simulink model "BR"  (R2020b)
settings: Solver=VariableStepAuto  StartTime=0.0  StopTime=10  RelTol=1e-3
undefined symbols (not defined in the file): U_nom
libraries: dspstat3 x12, powerlib x12, powerlib_meascontrol x3
settings Model: Creator=New-life  LastModifiedBy=New-life

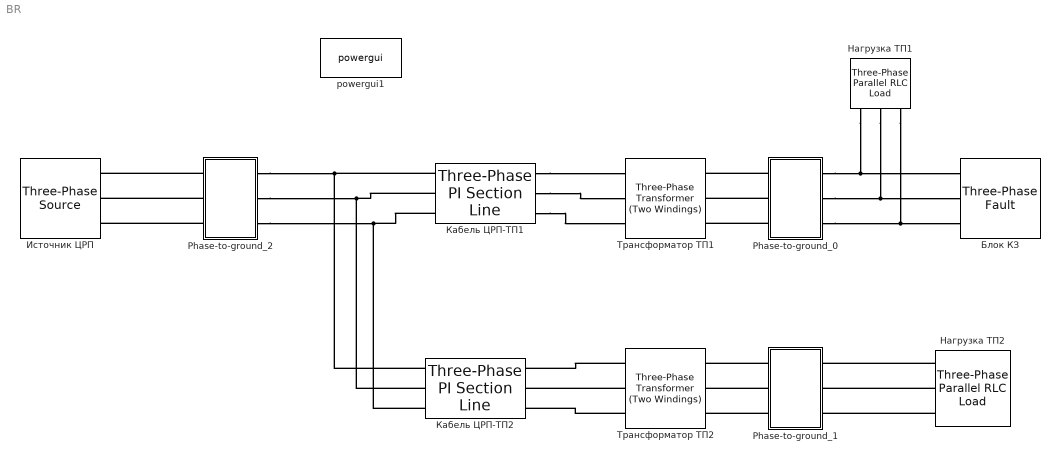
== system BR ==
  Phase-to-ground_0 : Subsystem
      settings: CopyFcn=|
      | % Получаем путь и имя нового (только что скопированного) блока
      | blockPath = gcb;
      | blockName = get_param(blockPath, 'Name');
      | 
      | % Ищем число в названии самой подсистемы (например, берем "2" из "Measure_2")
      | numStr = regexp(blockName, '\d+', 'match');
      | 
      | if ~isempty(numStr)
      |     newNum = numStr{end}; % Берем последнее найденное число
      | 
      |     % --- 1. Обновляем скрытые теги в Goto и From (радиочастоты) ---
      |     gotos = find_system(blockPath, 'LookUnderMasks', 'on', 'BlockType', 'Goto');
      |     froms = find_system(blockPath, 'LookUnderMasks', 'on', 'BlockType', 'From');
      | 
      |     for i = 1:length(gotos)
      |         oldTag = get_param(gotos{i}, 'GotoTag');
      |         set_param(gotos{i}, 'GotoTag', regexprep(oldTag, '\d+$', newNum));
      |     end
      |     for i = 1:length(froms)
      |         oldTag = get_param(froms{i}, 'GotoTag');
      |         set_param(froms{i}, 'GotoTag', regexprep(oldTag, '\d+$', newNum));
      |     end
      | 
      |     % --- 2. ПЕРЕИМЕНОВЫВАЕМ САМИ БЛОКИ (визуальные надписи UI0 -> UI1 и т.д.) ---
      |     % Ищем все элементы только внутри этой подсистемы
      |     internalBlocks = find_system(blockPath, 'SearchDepth', 1, 'LookUnderMasks', 'on');
      | 
      |     % Цикл начинаем с 2, так как 1-й элемент в списке - это сама папка подсистемы
      |     for i = 2:length(internalBlocks)
      |         oldName = get_param(internalBlocks{i}, 'Name');
      |         % Ищем цифру в конце имени и меняем на новую
      |         newName = regexprep(oldName, '\d+$', newNum);
      | 
      |         % Если имя изменилось, применяем его
      |         if ~strcmp(oldName, newName)
      |             try
      |                 set_param(internalBlocks{i}, 'Name', newName);
      |             catch
      |                 % Игнорируем ошибку, если вдруг такое имя уже случайно есть
      |             end
      |         end
      |     end
      | end
  Phase-to-ground_1 : Subsystem
      settings: CopyFcn=|
      | % Получаем путь и имя нового (только что скопированного) блока
      | blockPath = gcb;
      | blockName = get_param(blockPath, 'Name');
      | 
      | % Ищем число в названии самой подсистемы (например, берем "2" из "Measure_2")
      | numStr = regexp(blockName, '\d+', 'match');
      | 
      | if ~isempty(numStr)
      |     newNum = numStr{end}; % Берем последнее найденное число
      | 
      |     % --- 1. Обновляем скрытые теги в Goto и From (радиочастоты) ---
      |     gotos = find_system(blockPath, 'LookUnderMasks', 'on', 'BlockType', 'Goto');
      |     froms = find_system(blockPath, 'LookUnderMasks', 'on', 'BlockType', 'From');
      | 
      |     for i = 1:length(gotos)
      |         oldTag = get_param(gotos{i}, 'GotoTag');
      |         set_param(gotos{i}, 'GotoTag', regexprep(oldTag, '\d+$', newNum));
      |     end
      |     for i = 1:length(froms)
      |         oldTag = get_param(froms{i}, 'GotoTag');
      |         set_param(froms{i}, 'GotoTag', regexprep(oldTag, '\d+$', newNum));
      |     end
      | 
      |     % --- 2. ПЕРЕИМЕНОВЫВАЕМ САМИ БЛОКИ (визуальные надписи UI0 -> UI1 и т.д.) ---
      |     % Ищем все элементы только внутри этой подсистемы
      |     internalBlocks = find_system(blockPath, 'SearchDepth', 1, 'LookUnderMasks', 'on');
      | 
      |     % Цикл начинаем с 2, так как 1-й элемент в списке - это сама папка подсистемы
      |     for i = 2:length(internalBlocks)
      |         oldName = get_param(internalBlocks{i}, 'Name');
      |         % Ищем цифру в конце имени и меняем на новую
      |         newName = regexprep(oldName, '\d+$', newNum);
      | 
      |         % Если имя изменилось, применяем его
      |         if ~strcmp(oldName, newName)
      |             try
      |                 set_param(internalBlocks{i}, 'Name', newName);
      |             catch
      |                 % Игнорируем ошибку, если вдруг такое имя уже случайно есть
      |             end
      |         end
      |     end
      | end
  Phase-to-ground_2 : Subsystem
      settings: CopyFcn=|
      | % Получаем путь и имя нового (только что скопированного) блока
      | blockPath = gcb;
      | blockName = get_param(blockPath, 'Name');
      | 
      | % Ищем число в названии самой подсистемы (например, берем "2" из "Measure_2")
      | numStr = regexp(blockName, '\d+', 'match');
      | 
      | if ~isempty(numStr)
      |     newNum = numStr{end}; % Берем последнее найденное число
      | 
      |     % --- 1. Обновляем скрытые теги в Goto и From (радиочастоты) ---
      |     gotos = find_system(blockPath, 'LookUnderMasks', 'on', 'BlockType', 'Goto');
      |     froms = find_system(blockPath, 'LookUnderMasks', 'on', 'BlockType', 'From');
      | 
      |     for i = 1:length(gotos)
      |         oldTag = get_param(gotos{i}, 'GotoTag');
      |         set_param(gotos{i}, 'GotoTag', regexprep(oldTag, '\d+$', newNum));
      |     end
      |     for i = 1:length(froms)
      |         oldTag = get_param(froms{i}, 'GotoTag');
      |         set_param(froms{i}, 'GotoTag', regexprep(oldTag, '\d+$', newNum));
      |     end
      | 
      |     % --- 2. ПЕРЕИМЕНОВЫВАЕМ САМИ БЛОКИ (визуальные надписи UI0 -> UI1 и т.д.) ---
      |     % Ищем все элементы только внутри этой подсистемы
      |     internalBlocks = find_system(blockPath, 'SearchDepth', 1, 'LookUnderMasks', 'on');
      | 
      |     % Цикл начинаем с 2, так как 1-й элемент в списке - это сама папка подсистемы
      |     for i = 2:length(internalBlocks)
      |         oldName = get_param(internalBlocks{i}, 'Name');
      |         % Ищем цифру в конце имени и меняем на новую
      |         newName = regexprep(oldName, '\d+$', newNum);
      | 
      |         % Если имя изменилось, применяем его
      |         if ~strcmp(oldName, newName)
      |             try
      |                 set_param(internalBlocks{i}, 'Name', newName);
      |             catch
      |                 % Игнорируем ошибку, если вдруг такое имя уже случайно есть
      |             end
      |         end
      |     end
      | end
  powergui1 : powerlib/powergui  Priority=1  SimulationMode=Discrete  SampleTime=5e-5  frequency=60  Iterations=50  frequencyindice=50  Pbase=100e6  ErrMax=1e-4  UnitsV=kV  UnitsW=MW  buscounter=0  FunctionMessages=off  echomessages=off  EnableUseOfTLC=off  CurrentSourceSwitches=off  DisableSnubberDevices=off  DisableRonSwitches=off  DisableVfSwitches=off  DisplayEquations=off  AutomaticDiscreteSolvers=off  SolverType=Tustin/Backward Euler (TBE)  Interpol=off  ExternalGateDelay=off  methode=off  Ts=100  x0status=blocks  SPID=on  SwTol=0  HookPort=off  NonlinearTolerance=1e-4  nMaxIteration=100  ContinueOnMaxIteration=off  RestoreLinks=warning  ResistiveCurrentMeasurement=off  Frange=[0:2:500]  Ylog=off  Xlog=on  ShowGrid=off  save=off  variable=ZData  structure=0  ZoomFFT=off  StartTime=0.0  cycles=1  DisplayStyle=1  fundamental=60  FreqAxis=off  MaxFrequency=1000  frequencyindicesteady=1  RmsSteady=1  display=off
  Блок КЗ : powerlib/Elements/Three-Phase Fault  InitialStates=0  FaultA=on  FaultB=on  FaultC=on  GroundFault=off  SwitchTimes=T_fault  External=off  SwitchStatus=NaN  FaultResistance=0.001  GroundResistance=0.01  SnubberResistance=1e6  SnubberCapacitance=inf  Measurements=None
  Источник ЦРП : powerlib/Electrical Sources/Three-Phase Source  InternalConnection=Yg  VoltagePhases=off  Voltage=U_nom  PhaseAngle=0  Voltage_phases=[25e3 25e3 25e3]/sqrt(3)  PhaseAngles_phases=[0 -120 +120]  Frequency=50  NonIdealSource=on  SpecifyImpedance=on  Resistance=0.8929  Inductance=16.58e-3  ShortCircuitLevel=S_kz_sys  BaseVoltage=U_nom  XRratio=7  BusType=swing  Pref=10e3  Qref=0  Prefabc=[10e3, 10e3, 10e3]  Qrefabc=[0, 0, 0]  Qmin=-inf  Qmax=inf
  Кабель ЦРП-ТП1 : powerlib/Elements/Three-Phase PI Section Line  LConnTagsString=a|b|c  RConnTagsString=A|B|C  Length=L_cab1  Frequency=60  Resistances=[0.3 0.3]  Inductances=[0.637e-3 0.637e-3]  Capacitances=[0.3e-6 0.3e-6]
  Кабель ЦРП-ТП2 : powerlib/Elements/Three-Phase PI Section Line  LConnTagsString=a|b|c  RConnTagsString=A|B|C  Length=L_cab2  Frequency=60  Resistances=[0.3 0.3]  Inductances=[0.637e-3 0.637e-3]  Capacitances=[0.3e-6 0.3e-6]
  Нагрузка ТП1 : powerlib/Elements/Three-Phase Parallel RLC Load  LConnTagsString=A|B|C  Configuration=Y (grounded)  NominalVoltage=400  Vabc=[1e3 1e3 1e3]  Vabcp=[1e3 1e3 1e3]  NominalFrequency=50  UnbalancedPower=off  ActivePower=P_t1  InductivePower=Q_t1  CapacitivePower=0  Pabc=[10e3 9e3 11e3]  QLabc=[100 90 110]  QCabc=[100 90 110]  Pabcp=[10e3 9e3 11e3]  QLabcp=[100 90 110]  QCabcp=[100 90 110]  Measurements=None  LoadType=constant Z
  Нагрузка ТП2 : powerlib/Elements/Three-Phase Parallel RLC Load  LConnTagsString=A|B|C  Configuration=Y (grounded)  NominalVoltage=400  Vabc=[1e3 1e3 1e3]  Vabcp=[1e3 1e3 1e3]  NominalFrequency=50  UnbalancedPower=off  ActivePower=P_t2  InductivePower=Q_t2  CapacitivePower=0  Pabc=[10e3 9e3 11e3]  QLabc=[100 90 110]  QCabc=[100 90 110]  Pabcp=[10e3 9e3 11e3]  QLabcp=[100 90 110]  QCabcp=[100 90 110]  Measurements=None  LoadType=constant Z
  Трансформатор ТП1 : powerlib/Elements/Three-Phase Transformer (Two Windings)  Winding1Connection=Yg  Winding2Connection=Yg  CoreType=Three single-phase transformers  SetSaturation=off  Hysteresis=off  DataFile='hysteresis'  SetInitialFlux=off  Measurements=None  UNITS=pu  NominalPower=[630e3 50]  Winding1=[6000 0.005 0.02]  Winding2=[400 0.005 0.02]  Rm=500  Lm=500  L0=0.5  Saturation=[ 0,0 ; 0.0024,1.2 ; 1.0,1.52 ]  InitialFluxes=[ 0.8 , -0.8 , 0.7 ]  BreakLoop=off  DiscreteSolver=Trapezoidal iterative  DataType=off  TransfoNumber=1
  Трансформатор ТП2 : powerlib/Elements/Three-Phase Transformer (Two Windings)  Winding1Connection=Yg  Winding2Connection=Yg  CoreType=Three single-phase transformers  SetSaturation=off  Hysteresis=off  DataFile='hysteresis'  SetInitialFlux=off  Measurements=None  UNITS=pu  NominalPower=[630e3 50]  Winding1=[6000 0.005 0.02]  Winding2=[400 0.005 0.02]  Rm=500  Lm=500  L0=0.5  Saturation=[ 0,0 ; 0.0024,1.2 ; 1.0,1.52 ]  InitialFluxes=[ 0.8 , -0.8 , 0.7 ]  BreakLoop=off  DiscreteSolver=Trapezoidal iterative  DataType=off  TransfoNumber=1
  connections:
  Кабель ЦРП-ТП1/LConn1 -- Phase-to-ground_2/RConn1 -- Кабель ЦРП-ТП2/LConn1
  Кабель ЦРП-ТП1/LConn3 -- Phase-to-ground_2/RConn3 -- Кабель ЦРП-ТП2/LConn3
  Кабель ЦРП-ТП1/LConn2 -- Phase-to-ground_2/RConn2 -- Кабель ЦРП-ТП2/LConn2
  Кабель ЦРП-ТП1/RConn2 -- Трансформатор ТП1/LConn2
  Кабель ЦРП-ТП1/RConn3 -- Трансформатор ТП1/LConn3
  Кабель ЦРП-ТП1/RConn1 -- Трансформатор ТП1/LConn1
  Phase-to-ground_0/LConn2 -- Трансформатор ТП1/RConn2
  Phase-to-ground_0/LConn1 -- Трансформатор ТП1/RConn1
  Phase-to-ground_0/LConn3 -- Трансформатор ТП1/RConn3
  Phase-to-ground_0/RConn1 -- Нагрузка ТП1/LConn1 -- Блок КЗ/LConn1
  Phase-to-ground_0/RConn2 -- Нагрузка ТП1/LConn2 -- Блок КЗ/LConn2
  Phase-to-ground_0/RConn3 -- Блок КЗ/LConn3 -- Нагрузка ТП1/LConn3
  Нагрузка ТП2/LConn1 -- Phase-to-ground_1/RConn1
  Нагрузка ТП2/LConn2 -- Phase-to-ground_1/RConn2
  Нагрузка ТП2/LConn3 -- Phase-to-ground_1/RConn3
  Phase-to-ground_1/LConn1 -- Трансформатор ТП2/RConn1
  Phase-to-ground_1/LConn2 -- Трансформатор ТП2/RConn2
  Phase-to-ground_1/LConn3 -- Трансформатор ТП2/RConn3
  Трансформатор ТП2/LConn1 -- Кабель ЦРП-ТП2/RConn1
  Трансформатор ТП2/LConn2 -- Кабель ЦРП-ТП2/RConn2
  Трансформатор ТП2/LConn3 -- Кабель ЦРП-ТП2/RConn3
  Phase-to-ground_2/LConn3 -- Источник ЦРП/RConn3
  Phase-to-ground_2/LConn2 -- Источник ЦРП/RConn2
  Phase-to-ground_2/LConn1 -- Источник ЦРП/RConn1

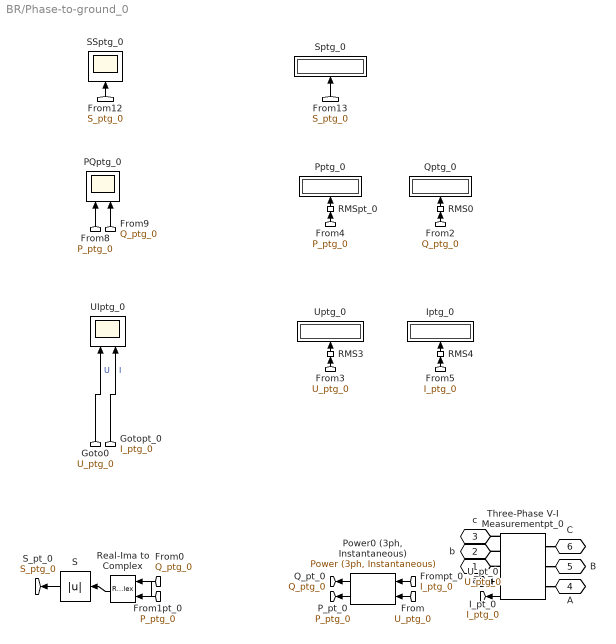
== system BR/Phase-to-ground_0 ==
  Iptg_0 : Display
      settings: Format=bank
  PQptg_0 : Scope  NumInputPorts=2
  "Power0 (3ph, Instantaneous)" : powerlib_meascontrol/Measurements/Power (3ph, Instantaneous)
  Pptg_0 : Display
      settings: Format=bank
  Qptg_0 : Display
      settings: Format=bank
  RMS0 : dspstat3/RMS  run=off  directionMode=Each column  dimension=1  InputProcessing=Columns as channels (frame based)  reset_popup=None
  RMS3 : dspstat3/RMS  run=off  directionMode=Each column  dimension=1  InputProcessing=Columns as channels (frame based)  reset_popup=None
  RMS4 : dspstat3/RMS  run=off  directionMode=Each column  dimension=1  InputProcessing=Columns as channels (frame based)  reset_popup=None
  RMSpt_0 : dspstat3/RMS  run=off  directionMode=Each column  dimension=1  InputProcessing=Columns as channels (frame based)  reset_popup=None
  Real-Ima to Complex : RealImagToComplex
  S : Abs
  SSptg_0 : Scope
  Sptg_0 : Display
      settings: Format=bank
  Three-Phase V-I Measurementpt_0 : powerlib/Measurements/Three-Phase V-I Measurement  VoltageMeasurement=phase-to-ground  SetLabelV=off  LabelV=Vabc  Vpu=off  VpuLL=off  CurrentMeasurement=yes  SetLabelI=off  LabelI=Iabc  Ipu=off  Pbase=100e6  Vbase=500e3  OutputType=Complex  PhasorSimulation=off  PSBequivalent=0
  UIptg_0 : Scope  NumInputPorts=2
  Uptg_0 : Display
      settings: Format=bank
  a : PMIOPort  Side=Right
  b : PMIOPort  Port=2  Side=Right
  c : PMIOPort  Port=3  Side=Right
  A : PMIOPort  Port=4  Side=Left
  B : PMIOPort  Port=5  Side=Left
  C : PMIOPort  Port=6  Side=Left
  tag scope: I_ptg_0=global, P_ptg_0=global, Q_ptg_0=global, S_ptg_0=global, U_ptg_0=global
  wires:
  S/1 -> [S_ptg_0]
  Real-Ima to Complex/1 -> S/1
  [S_ptg_0] -> Sptg_0/1
  [S_ptg_0] -> SSptg_0/1
  [P_ptg_0] -> RMSpt_0/1
  RMSpt_0/1 -> Pptg_0/1
  RMS0/1 -> Qptg_0/1
  [U_ptg_0] -> RMS3/1
  RMS3/1 -> Uptg_0/1
  [P_ptg_0] -> Real-Ima to Complex/1
  [Q_ptg_0] -> RMS0/1
  [I_ptg_0] -> RMS4/1
  RMS4/1 -> Iptg_0/1
  [P_ptg_0] -> PQptg_0/1
  [I_ptg_0] -> UIptg_0/2  "I"
  Three-Phase V-I Measurementpt_0/1 -> [U_ptg_0]
  [Q_ptg_0] -> Real-Ima to Complex/2
  Three-Phase V-I Measurementpt_0/2 -> [I_ptg_0]
  [U_ptg_0] -> "Power0 (3ph, Instantaneous)"/1
  [I_ptg_0] -> "Power0 (3ph, Instantaneous)"/2
  [Q_ptg_0] -> PQptg_0/2
  "Power0 (3ph, Instantaneous)"/2 -> [Q_ptg_0]
  "Power0 (3ph, Instantaneous)"/1 -> [P_ptg_0]
  [U_ptg_0] -> UIptg_0/1  "U"
  connections:
  Three-Phase V-I Measurementpt_0/LConn1 -- A/RConn1
  Three-Phase V-I Measurementpt_0/RConn1 -- a/RConn1
  Three-Phase V-I Measurementpt_0/LConn2 -- B/RConn1
  Three-Phase V-I Measurementpt_0/LConn3 -- C/RConn1
  Three-Phase V-I Measurementpt_0/RConn3 -- c/RConn1
  Three-Phase V-I Measurementpt_0/RConn2 -- b/RConn1

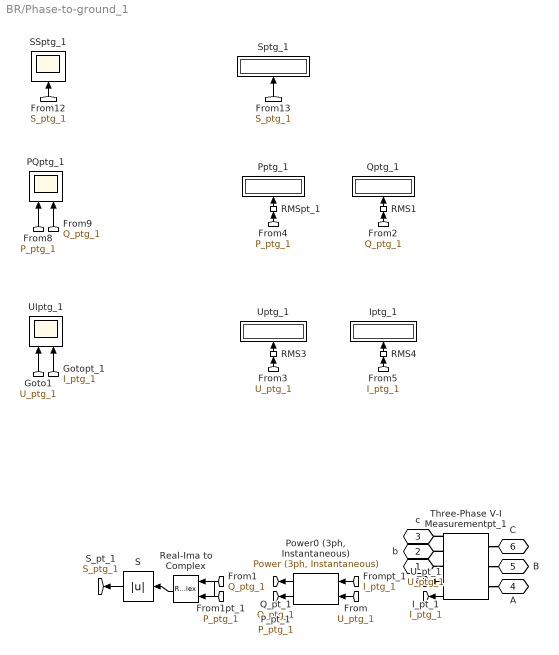
== system BR/Phase-to-ground_1 ==
  Iptg_1 : Display
      settings: Format=bank
  PQptg_1 : Scope  NumInputPorts=2
  "Power0 (3ph, Instantaneous)" : powerlib_meascontrol/Measurements/Power (3ph, Instantaneous)
  Pptg_1 : Display
      settings: Format=bank
  Qptg_1 : Display
      settings: Format=bank
  RMS1 : dspstat3/RMS  run=off  directionMode=Each column  dimension=1  InputProcessing=Columns as channels (frame based)  reset_popup=None
  RMS3 : dspstat3/RMS  run=off  directionMode=Each column  dimension=1  InputProcessing=Columns as channels (frame based)  reset_popup=None
  RMS4 : dspstat3/RMS  run=off  directionMode=Each column  dimension=1  InputProcessing=Columns as channels (frame based)  reset_popup=None
  RMSpt_1 : dspstat3/RMS  run=off  directionMode=Each column  dimension=1  InputProcessing=Columns as channels (frame based)  reset_popup=None
  Real-Ima to Complex : RealImagToComplex
  S : Abs
  SSptg_1 : Scope
  Sptg_1 : Display
      settings: Format=bank
  Three-Phase V-I Measurementpt_1 : powerlib/Measurements/Three-Phase V-I Measurement  VoltageMeasurement=phase-to-ground  SetLabelV=off  LabelV=Vabc  Vpu=off  VpuLL=off  CurrentMeasurement=yes  SetLabelI=off  LabelI=Iabc  Ipu=off  Pbase=100e6  Vbase=500e3  OutputType=Complex  PhasorSimulation=off  PSBequivalent=0
  UIptg_1 : Scope  NumInputPorts=2
  Uptg_1 : Display
      settings: Format=bank
  a : PMIOPort  Side=Right
  b : PMIOPort  Port=2  Side=Right
  c : PMIOPort  Port=3  Side=Right
  A : PMIOPort  Port=4  Side=Left
  B : PMIOPort  Port=5  Side=Left
  C : PMIOPort  Port=6  Side=Left
  tag scope: I_ptg_1=global, P_ptg_1=global, Q_ptg_1=global, S_ptg_1=global, U_ptg_1=global
  wires:
  [Q_ptg_1] -> PQptg_1/2
  "Power0 (3ph, Instantaneous)"/1 -> [P_ptg_1]
  "Power0 (3ph, Instantaneous)"/2 -> [Q_ptg_1]
  [I_ptg_1] -> "Power0 (3ph, Instantaneous)"/2
  [U_ptg_1] -> "Power0 (3ph, Instantaneous)"/1
  Three-Phase V-I Measurementpt_1/2 -> [I_ptg_1]
  [Q_ptg_1] -> Real-Ima to Complex/2
  Three-Phase V-I Measurementpt_1/1 -> [U_ptg_1]
  [I_ptg_1] -> UIptg_1/2
  [P_ptg_1] -> PQptg_1/1
  [U_ptg_1] -> UIptg_1/1
  RMS4/1 -> Iptg_1/1
  [I_ptg_1] -> RMS4/1
  [Q_ptg_1] -> RMS1/1
  [P_ptg_1] -> Real-Ima to Complex/1
  RMS3/1 -> Uptg_1/1
  [U_ptg_1] -> RMS3/1
  RMS1/1 -> Qptg_1/1
  RMSpt_1/1 -> Pptg_1/1
  [P_ptg_1] -> RMSpt_1/1
  [S_ptg_1] -> SSptg_1/1
  [S_ptg_1] -> Sptg_1/1
  Real-Ima to Complex/1 -> S/1
  S/1 -> [S_ptg_1]
  connections:
  Three-Phase V-I Measurementpt_1/RConn2 -- b/RConn1
  Three-Phase V-I Measurementpt_1/RConn3 -- c/RConn1
  Three-Phase V-I Measurementpt_1/LConn3 -- C/RConn1
  Three-Phase V-I Measurementpt_1/LConn2 -- B/RConn1
  Three-Phase V-I Measurementpt_1/RConn1 -- a/RConn1
  Three-Phase V-I Measurementpt_1/LConn1 -- A/RConn1

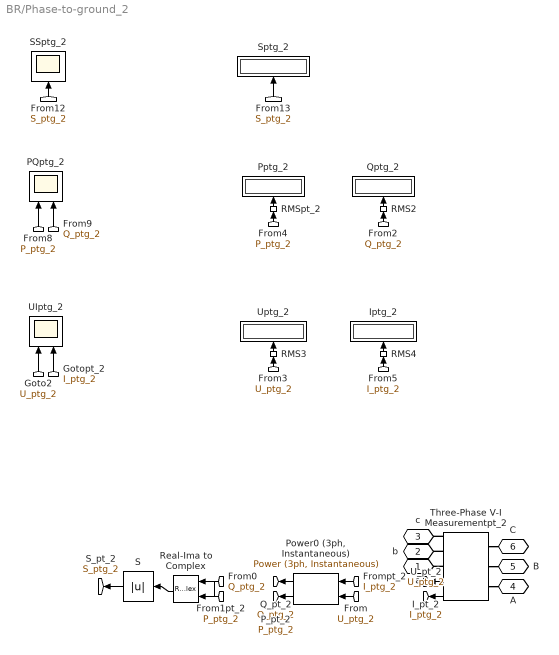
== system BR/Phase-to-ground_2 ==
  Iptg_2 : Display
      settings: Format=bank
  PQptg_2 : Scope  NumInputPorts=2
  "Power0 (3ph, Instantaneous)" : powerlib_meascontrol/Measurements/Power (3ph, Instantaneous)
  Pptg_2 : Display
      settings: Format=bank
  Qptg_2 : Display
      settings: Format=bank
  RMS2 : dspstat3/RMS  run=off  directionMode=Each column  dimension=1  InputProcessing=Columns as channels (frame based)  reset_popup=None
  RMS3 : dspstat3/RMS  run=off  directionMode=Each column  dimension=1  InputProcessing=Columns as channels (frame based)  reset_popup=None
  RMS4 : dspstat3/RMS  run=off  directionMode=Each column  dimension=1  InputProcessing=Columns as channels (frame based)  reset_popup=None
  RMSpt_2 : dspstat3/RMS  run=off  directionMode=Each column  dimension=1  InputProcessing=Columns as channels (frame based)  reset_popup=None
  Real-Ima to Complex : RealImagToComplex
  S : Abs
  SSptg_2 : Scope
  Sptg_2 : Display
      settings: Format=bank
  Three-Phase V-I Measurementpt_2 : powerlib/Measurements/Three-Phase V-I Measurement  VoltageMeasurement=phase-to-ground  SetLabelV=off  LabelV=Vabc  Vpu=off  VpuLL=off  CurrentMeasurement=yes  SetLabelI=off  LabelI=Iabc  Ipu=off  Pbase=100e6  Vbase=500e3  OutputType=Complex  PhasorSimulation=off  PSBequivalent=0
  UIptg_2 : Scope  NumInputPorts=2
  Uptg_2 : Display
      settings: Format=bank
  a : PMIOPort  Side=Right
  b : PMIOPort  Port=2  Side=Right
  c : PMIOPort  Port=3  Side=Right
  A : PMIOPort  Port=4  Side=Left
  B : PMIOPort  Port=5  Side=Left
  C : PMIOPort  Port=6  Side=Left
  tag scope: I_ptg_2=global, P_ptg_2=global, Q_ptg_2=global, S_ptg_2=global, U_ptg_2=global
  wires:
  [Q_ptg_2] -> PQptg_2/2
  "Power0 (3ph, Instantaneous)"/1 -> [P_ptg_2]
  "Power0 (3ph, Instantaneous)"/2 -> [Q_ptg_2]
  [I_ptg_2] -> "Power0 (3ph, Instantaneous)"/2
  [U_ptg_2] -> "Power0 (3ph, Instantaneous)"/1
  Three-Phase V-I Measurementpt_2/2 -> [I_ptg_2]
  [Q_ptg_2] -> Real-Ima to Complex/2
  Three-Phase V-I Measurementpt_2/1 -> [U_ptg_2]
  [I_ptg_2] -> UIptg_2/2
  [P_ptg_2] -> PQptg_2/1
  [U_ptg_2] -> UIptg_2/1
  RMS4/1 -> Iptg_2/1
  [I_ptg_2] -> RMS4/1
  [Q_ptg_2] -> RMS2/1
  [P_ptg_2] -> Real-Ima to Complex/1
  RMS3/1 -> Uptg_2/1
  [U_ptg_2] -> RMS3/1
  RMS2/1 -> Qptg_2/1
  RMSpt_2/1 -> Pptg_2/1
  [P_ptg_2] -> RMSpt_2/1
  [S_ptg_2] -> SSptg_2/1
  [S_ptg_2] -> Sptg_2/1
  Real-Ima to Complex/1 -> S/1
  S/1 -> [S_ptg_2]
  connections:
  Three-Phase V-I Measurementpt_2/RConn2 -- b/RConn1
  Three-Phase V-I Measurementpt_2/RConn3 -- c/RConn1
  Three-Phase V-I Measurementpt_2/LConn3 -- C/RConn1
  Three-Phase V-I Measurementpt_2/LConn2 -- B/RConn1
  Three-Phase V-I Measurementpt_2/RConn1 -- a/RConn1
  Three-Phase V-I Measurementpt_2/LConn1 -- A/RConn1
